simulink model "ETS"  (R2018a)
settings: configuration reference "cs_ert" (kept outside this file)
settings Model: DataDictionary=ETS.sldd  Creator=zhoutinglin  LastModifiedBy=zhoutinglin

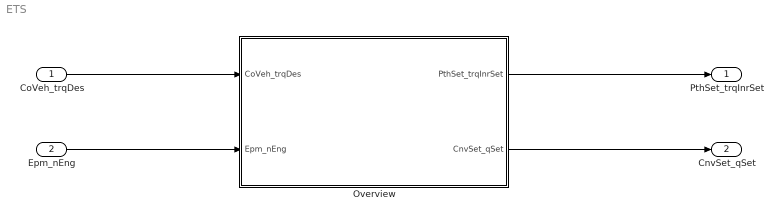
== system ETS ==
  CoVeh_trqDes : Inport
  Epm_nEng : Inport  Port=2
  Overview : Subsystem
  PthSet_trqInrSet : Outport
  CnvSet_qSet : Outport  Port=2
  wires:
  CoVeh_trqDes/1 -> Overview/1(CoVeh_trqDes)
  Epm_nEng/1 -> Overview/2(Epm_nEng)
  Overview/1(PthSet_trqInrSet) -> PthSet_trqInrSet/1
  Overview/2(CnvSet_qSet) -> CnvSet_qSet/1

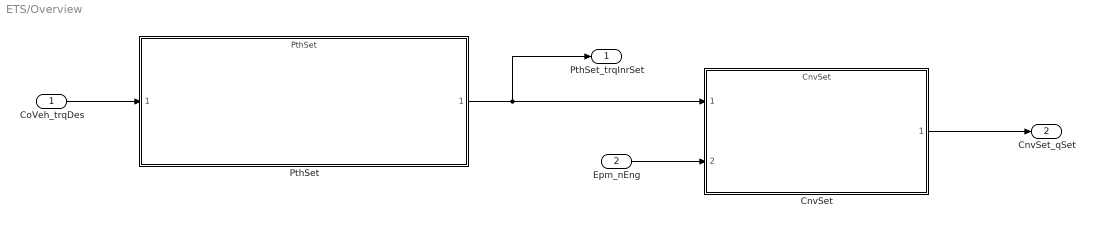
== system ETS/Overview ==
  CoVeh_trqDes : Inport
  Epm_nEng : Inport  Port=2
  CnvSet : ModelReference  ModelNameDialog=CnvSet  SimulationMode=Normal  ModelReferenceVersion=1.2
  PthSet : ModelReference  ModelNameDialog=PthSet  SimulationMode=Normal  ModelReferenceVersion=1.2
  PthSet_trqInrSet : Outport
  CnvSet_qSet : Outport  Port=2
  wires:
  PthSet/1 -> CnvSet/1, PthSet_trqInrSet/1
  CoVeh_trqDes/1 -> PthSet/1
  Epm_nEng/1 -> CnvSet/2
  CnvSet/1 -> CnvSet_qSet/1
